simulink model "HW02_feedforward_control_2023_1106"  (R2023a)
settings: Solver=VariableStepAuto  StartTime=0.0  StopTime=50  RelTol=1e-3
libraries: slpidlib x1
settings Model: Creator=YYlab_05  LastModifiedBy=YYlab_05

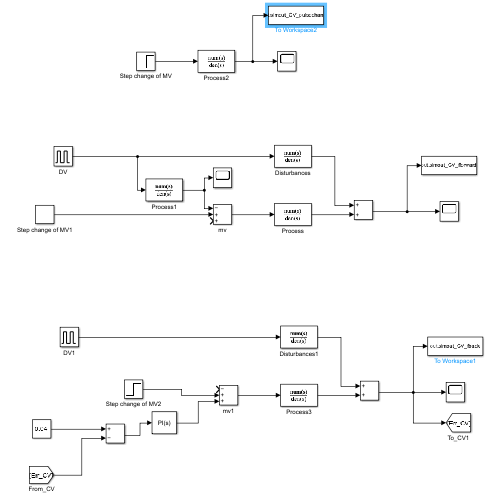
[thumbnail: Simulink's stored preview of the top-level diagram]
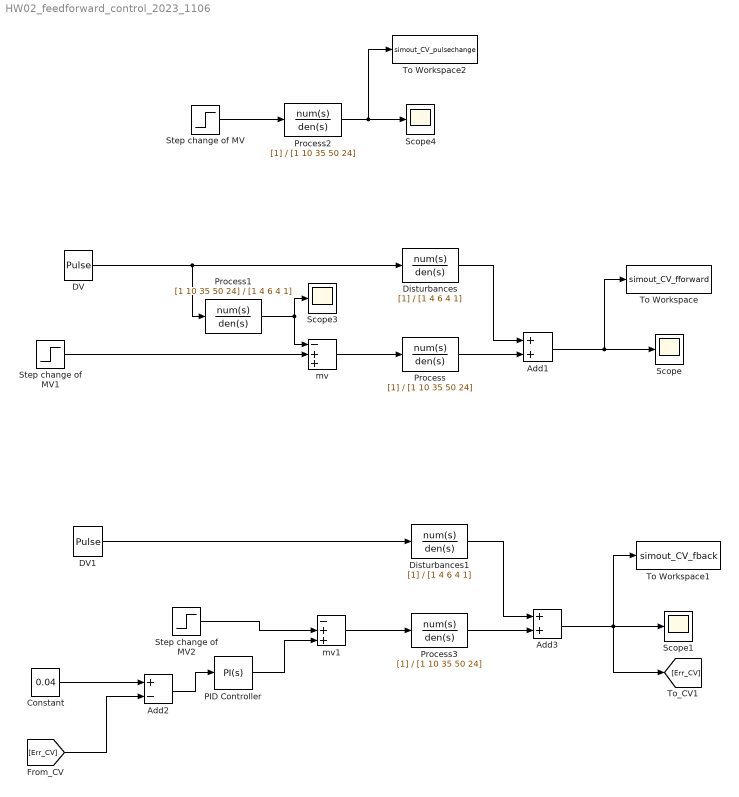
== system HW02_feedforward_control_2023_1106 ==
  Add1 : Sum
  Add2 : Sum  Inputs=+-
  Add3 : Sum
  Constant : Constant  Value=0.04
  DV : DiscretePulseGenerator  PulseType=Time based  Period=5  PulseWidth=20
  DV1 : DiscretePulseGenerator  PulseType=Time based  Period=5  PulseWidth=20
  Disturbances : TransferFcn  Denominator=[1 4 6 4 1]
  Disturbances1 : TransferFcn  Denominator=[1 4 6 4 1]
  PID Controller : slpidlib/PID Controller  Controller=PI  Form=Parallel  TimeDomain=Continuous-time  UseExternalTs=off  SampleTime=-1  IntegratorMethod=Forward Euler  FilterMethod=Forward Euler  ControllerParametersSource=internal  P=0.9/0.036  I=9/0.3  UseKiTs=on  D=0  N=100  UseFilter=on  TunerSelectOption=Transfer Function Based (PID Tuner App)  InitialConditionSource=internal  InitialConditionForIntegrator=0  InitialConditionForFilter=0  DifferentiatorICPrevScaledInput=0  ExternalReset=none  TrackingMode=off  Kt=1  LimitOutput=off  SatLimitsSource=internal  UpperSaturationLimit=inf  LowerSaturationLimit=-inf  LinearizeAsGain=on  AntiWindupMode=none  Kb=1  LimitIntegrator=off  UpperIntegratorSaturationLimit=inf  LowerIntegratorSaturationLimit=-inf  POutMin=[]  POutMax=[]  IOutMin=[]  IOutMax=[]  DOutMin=[]  DOutMax=[]  NOutMin=[]  NOutMax=[]  SumOutMin=[]  SumOutMax=[]  SaturationOutMin=[]  SaturationOutMax=[]  PParamMin=[]  PParamMax=[]  IParamMin=[]  IParamMax=[]  DParamMin=[]  DParamMax=[]  NParamMin=[]  NParamMax=[]  KbParamMin=[]  KbParamMax=[]  KtParamMin=[]  KtParamMax=[]  KbOutMin=[]  KbOutMax=[]  KtOutMin=[]  KtOutMax=[]  IntegratorOutMin=[]  IntegratorOutMax=[]  FilterOutMin=[]  FilterOutMax=[]  SumI1OutMin=[]  SumI1OutMax=[]  SumI2OutMin=[]  SumI2OutMax=[]  SumI3OutMin=[]  SumI3OutMax=[]  SumI4OutMin=[]  SumI4OutMax=[]  SumDOutMin=[]  SumDOutMax=[]  DifferentiatorOutMin=[]  DifferentiatorOutMax=[]  FilterDiffOutCoefMin=[]  FilterDiffOutCoefMax=[]  ReciprocalOutMin=[]  ReciprocalOutMax=[]  SumDenOutMin=[]  SumDenOutMax=[]  SumNumOutMin=[]  SumNumOutMax=[]  DivideOutMin=[]  DivideOutMax=[]  UdiffTsProdOutMin=[]  UdiffTsProdOutMax=[]  NTsProdOutMin=[]  NTsProdOutMax=[]  UintegralTsProdOutMin=[]  UintegralTsProdOutMax=[]  UngainTsProdOutMin=[]  UngainTsProdOutMax=[]  ClampingZeroOutDataTypeStr=Inherit: Inherit via back propagation  ClampingZeroOutMin=[]  ClampingZeroOutMax=[]  FilterDenConstantOutDataTypeStr=Inherit: Inherit via back propagation  FilterDenConstantOutMin=[]  FilterDenConstantOutMax=[]  PCopyOutDataTypeStr=Inherit: Inherit via back propagation  PCopyOutMin=[]  PCopyOutMax=[]  NCopyOutDataTypeStr=Inherit: Inherit via back propagation  NCopyOutMin=[]  NCopyOutMax=[]  IntegratorContinuousStateAttributes=''  IntegratorStateMustResolveToSignalObject=off  IntegratorRTWStateStorageClass=Auto  FilterContinuousStateAttributes=''  FilterStateMustResolveToSignalObject=off  FilterRTWStateStorageClass=Auto  ParallelPVariant=InternalParameters  IdealPVariant=Disabled  IVariant=InternalParameters  DVariant=Disabled  IntegratorVariant=Continuous  SatVariant=Disabled  AWVariant=Passthrough  PCopyVariant=Disabled  TRVariant=Disabled  FdbkBlocksVariant=Forward  IdealPFdbkVariant=Disabled  SatFdbkVariant=Disabled  DerivativeFilterVariant=Disabled  NVariant=Disabled  NCopyVariant=Disabled_SignalSpec  FilterICVariant=Disabled  IntegratorICVariant=InternalICs  ExternalResetVariant=Disabled  TRSumVariant=Passthrough  SumFdbkVariant=Disabled  SumVariant=Sum_PI  TsampFilterVariant=InternalTs  TsampNgainVariant=Passthrough  TsampIntegralVariant=Disabled_SignalSpec  ExternalSaturationOutDataTypeStr=Inherit: Same as second input
  Process : TransferFcn  Denominator=[1 10 35 50 24]
  Process1 : TransferFcn  Numerator=[1 10 35 50 24]  Denominator=[1 4 6 4 1]
  Process2 : TransferFcn  Denominator=[1 10 35 50 24]
  Process3 : TransferFcn  Denominator=[1 10 35 50 24]
  Scope{,1,3..4} (4 alike) : Scope
  Step change of MV : Step  SampleTime=0
  Step change of MV1 : Step  SampleTime=0
  Step change of MV2 : Step  SampleTime=0
  To Workspace : ToWorkspace  VariableName=simout_CV_fforward  SaveFormat=Timeseries  SampleTime=-1
  To Workspace1 : ToWorkspace  VariableName=simout_CV_fback  SaveFormat=Timeseries  SampleTime=-1
  To Workspace2 : ToWorkspace  VariableName=simout_CV_pulsechange  SaveFormat=Timeseries  SampleTime=-1
  mv : Sum  Inputs=-++
  mv1 : Sum  Inputs=-++
  wires:
  mv/1 -> Process/1
  Process/1 -> Add1/2
  DV/1 -> Process1/1, Disturbances/1
  Process1/1 -> Scope3/1, mv/1
  Add1/1 -> Scope/1, To Workspace/1
  Add2/1 -> PID Controller/1
  Step change of MV/1 -> Process2/1
  [Err_CV] -> Add2/2
  Disturbances/1 -> Add1/1
  Step change of MV1/1 -> mv/2
  Disturbances1/1 -> Add3/1
  Step change of MV2/1 -> mv1/2
  DV1/1 -> Disturbances1/1
  Process3/1 -> Add3/2
  Add3/1 -> [Err_CV], Scope1/1, To Workspace1/1
  mv1/1 -> Process3/1
  Constant/1 -> Add2/1
  PID Controller/1 -> mv1/3
  Process2/1 -> To Workspace2/1, Scope4/1
